simulink model "Engine_Control_Complex"  (R2018a)
settings: Solver=VariableStepAuto  StartTime=0.0  StopTime=20  MaxStep=0.01  RelTol=1e-9
settings Model: Creator=rahul  LastModifiedBy=rahul

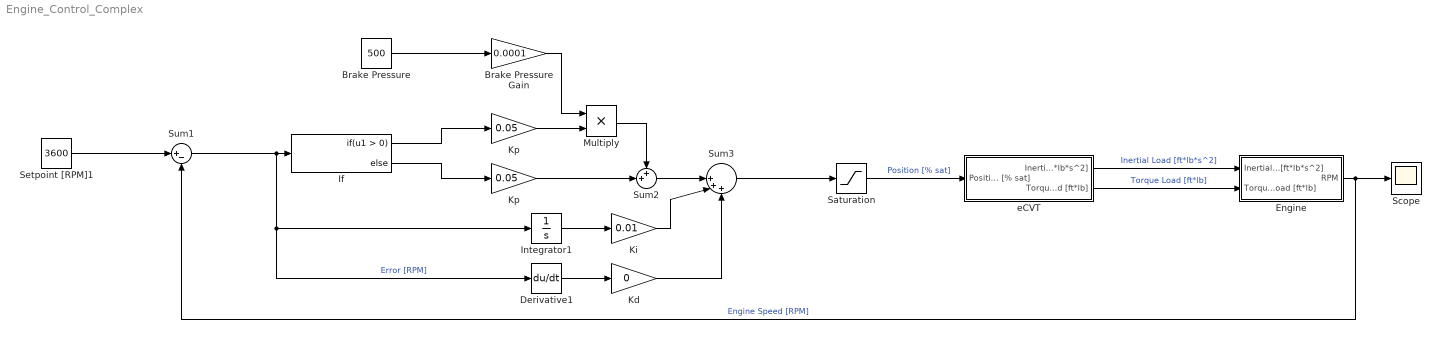
== system Engine_Control_Complex ==
  Brake Pressure : Constant  Value=500
  Brake Pressure Gain : Gain  Gain=0.0001
  Derivative1 : Derivative
  Engine : Subsystem
  "If " : If
  Integrator1 : Integrator
  Kd : Gain  Gain=0
  Ki : Gain  Gain=0.01
  Kp : Gain  Gain=0.05
  "Kp " : Gain  Gain=0.05
  "Multiply " : Product
  Saturation : Saturate  UpperLimit=1  LowerLimit=0
  Scope : Scope
  Setpoint [RPM]1 : Constant  Value=3600
  Sum1 : Sum  Inputs=|+-
  Sum2 : Sum  Inputs=++|
  Sum3 : Sum  Inputs=||+++
  eCVT : Subsystem
  wires:
  eCVT/1(Inertial Load [ft*lb*s^2]) -> Engine/1(Inertial Load [ft*lb*s^2])  "Inertial Load [ft*lb*s^2]"
  eCVT/2(Torque Load [ft*lb]) -> Engine/2(Torque Load [ft*lb])  "Torque Load [ft*lb]"
  "Kp "/1 -> "Multiply "/2
  "If "/2 -> Kp/1
  Brake Pressure Gain/1 -> "Multiply "/1
  Kp/1 -> Sum2/2
  Sum3/1 -> Saturation/1
  "If "/1 -> "Kp "/1
  Brake Pressure/1 -> Brake Pressure Gain/1
  Sum1/1 -> Derivative1/1, Integrator1/1, "If "/1  "Error [RPM]"
  Derivative1/1 -> Kd/1
  Sum2/1 -> Sum3/1
  Ki/1 -> Sum3/2
  Setpoint [RPM]1/1 -> Sum1/1
  Integrator1/1 -> Ki/1
  "Multiply "/1 -> Sum2/1
  Kd/1 -> Sum3/3
  Saturation/1 -> eCVT/1(Position [% sat])  "Position [% sat]"
  Engine/1(RPM) -> Scope/1, Sum1/2  "Engine Speed [RPM]"

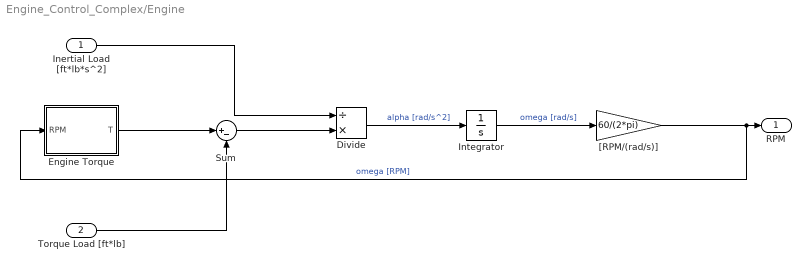
== system Engine_Control_Complex/Engine ==
  Inertial Load [ft*lb*s^2] : Inport
  Torque Load [ft*lb] : Inport  Port=2
  Divide : Product  Inputs=/*
  Engine Torque : MATLAB Function  TreatAsAtomicUnit=on
  "Integrator " : Integrator  InitialCondition=3000*(2*pi)/60
  Sum : Sum  Inputs=|+-
  "[RPM/(rad/s)]" : Gain  Gain=60/(2*pi)
  RPM : Outport
  wires:
  "Integrator "/1 -> "[RPM/(rad/s)]"/1  "omega [rad/s]"
  "[RPM/(rad/s)]"/1 -> Engine Torque/1(RPM), RPM/1  "omega [RPM]"
  Divide/1 -> "Integrator "/1  "alpha [rad/s^2]"
  Engine Torque/1(T) -> Sum/1
  Torque Load [ft*lb]/1 -> Sum/2
  Sum/1 -> Divide/2
  Inertial Load [ft*lb*s^2]/1 -> Divide/1

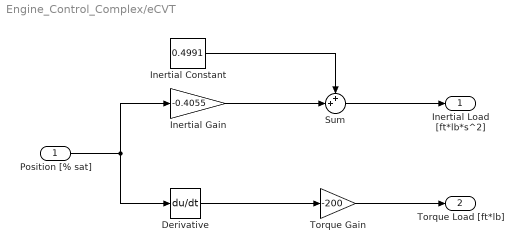
== system Engine_Control_Complex/eCVT ==
  Position [% sat] : Inport
  "Derivative " : Derivative
  Inertial Constant : Constant  Value=0.4991
  Inertial Gain : Gain  Gain=-0.4055
  Sum : Sum  Inputs=++|
  Torque Gain : Gain  Gain=-200
  Inertial Load [ft*lb*s^2] : Outport
  Torque Load [ft*lb] : Outport  Port=2
  wires:
  Position [% sat]/1 -> Inertial Gain/1, "Derivative "/1
  Sum/1 -> Inertial Load [ft*lb*s^2]/1
  Inertial Gain/1 -> Sum/2
  Inertial Constant/1 -> Sum/1
  "Derivative "/1 -> Torque Gain/1
  Torque Gain/1 -> Torque Load [ft*lb]/1

== matlab function Engine_Control_Complex/Engine/Engine Torque ==
  data: RPM input; T output
function T = fcn(RPM)

% RPM < 1750
if RPM < 1750
    T = 0;

% 1750 < RPM < 3800
elseif RPM < 3600
    % BSM19 Engine HP vs. RPM Equation  (3rd Order)
    HP = - 2.874 * 10^-10 * RPM.^3 ...
         + 1.781 * 10^-06 * RPM.^2 ...
         - 6.842 * 10^-04 * RPM.^1 ...
         + 1.719 * 10^000 * RPM.^0;

    % Torque = Power / Angular Velocity
    T = HP ./ (RPM*2*pi) * 33000;

% 3600 < RPM < 3800
elseif RPM < 3800
    % Linearized Governor
    T = -0.065 * RPM + 247;

% RPM > 3800
else
    T = 0;

end
